simulink model "Rect_fed_NL_load_Single_phase_active_filter"  (R2024b)
settings: Solver=ode4  StartTime=0.0  StopTime=1  FixedStep=1e-6  RelTol=1e-3
undefined symbols (not defined in the file or in its folder): THD
libraries: spsCurrentMeasurementLib x5, spsSeriesRLCBranchLib x5, spsDiodeLib x4, spsMosfetLib x4, spsVoltageMeasurementLib x3, slpidlib x2, spsACVoltageSourceLib x1, spspowerguiLib x1
settings Model: Creator=adity  LastModifiedBy=adity

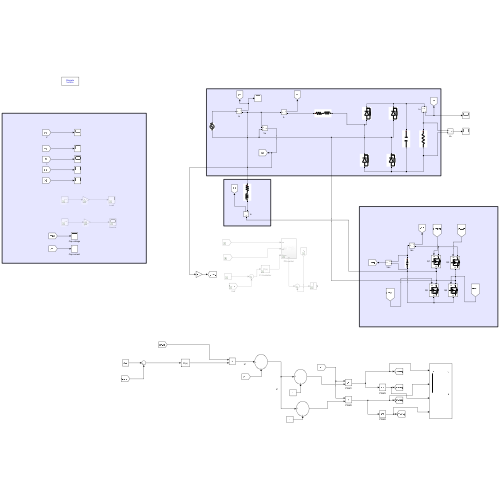
[thumbnail: Simulink's stored preview of the top-level diagram]
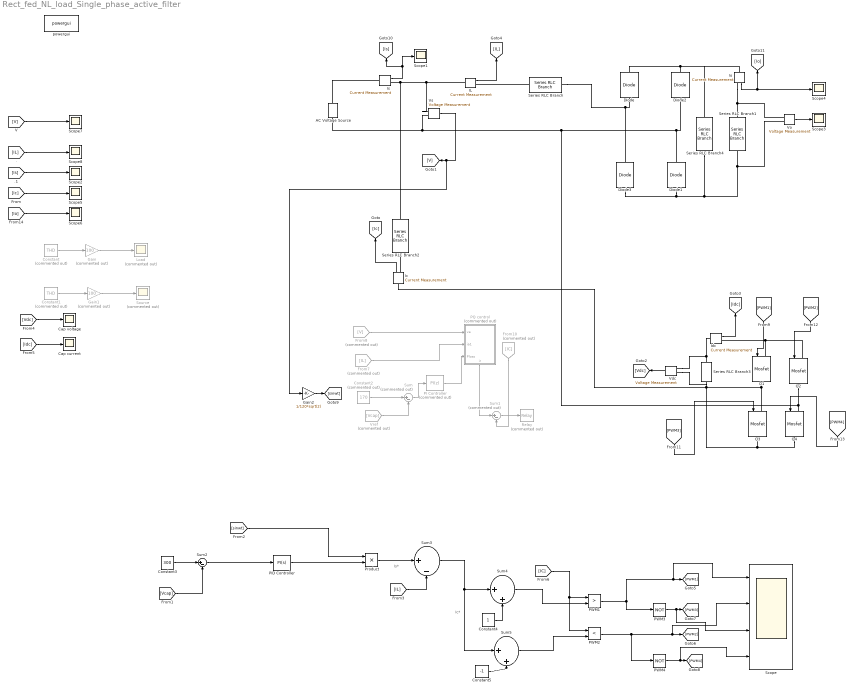
== system Rect_fed_NL_load_Single_phase_active_filter ==
  note: Ic*
  note: Is*
  AC Voltage Source : spsACVoltageSourceLib/AC Voltage Source  Amplitude=120*sqrt(2)  Phase=0  Frequency=60  SampleTime=0  Measurements=None  BusType=swing  Pref=10e3  Qref=0  Qmin=-inf  Qmax=+inf
  Cap current : Scope
  Cap voltage : Scope
  Constant : Constant  Commented=on  Value=THD
  Constant1 : Constant  Commented=on  Value=THD
  Constant2 : Constant  Commented=on  Value=170
  Constant3 : Constant  Value=300
  Constant4 : Constant
  Constant5 : Constant  Value=-1
  Diode{,1..3} (4 alike) : spsDiodeLib/Diode  Ron=0.001  Lon=0  Vf=0.8  IC=0  UseSnubber=0  Rs=500  Cs=250e-9  Measurements=off
  From10 : From  Commented=on  GotoTag=IC
  From7 : From  Commented=on  GotoTag=IL
  From8 : From  Commented=on  GotoTag=V
  Gain : Gain  Commented=on  Gain=100
  Gain1 : Gain  Commented=on  Gain=100
  Gain2 : Gain  Gain=1/120*sqrt(2)
  IL : spsCurrentMeasurementLib/Current Measurement  PhasorSimulation=off  OutputType=Complex  PSBequivalent=0
  Ic : spsCurrentMeasurementLib/Current Measurement  PhasorSimulation=off  OutputType=Complex  PSBequivalent=0
  Idc : spsCurrentMeasurementLib/Current Measurement  PhasorSimulation=off  OutputType=Complex  PSBequivalent=0
  Io : spsCurrentMeasurementLib/Current Measurement  PhasorSimulation=off  OutputType=Complex  PSBequivalent=0
  Is : spsCurrentMeasurementLib/Current Measurement  PhasorSimulation=off  OutputType=Complex  PSBequivalent=0
  Load : Scope  Commented=on
  PI Controller : slpidlib/PID Controller  Commented=on  Controller=PI  Form=Parallel  TimeDomain=Discrete-time  UseExternalTs=off  SampleTime=-1  IntegratorMethod=Forward Euler  FilterMethod=Forward Euler  ControllerParametersSource=internal  P=0.425  I=0.4  UseKiTs=off  D=0  UseExternalDerivativeSource=off  N=100  UseFilter=on  TunerSelectOption=Transfer Function Based (PID Tuner App)  InitialConditionSource=internal  InitialConditionForIntegrator=0  InitialConditionForFilter=0  DifferentiatorICPrevScaledInput=0  ExternalReset=none  TrackingMode=off  Kt=1  LimitOutput=off  SatLimitsSource=internal  UpperSaturationLimit=inf  LowerSaturationLimit=-inf  LinearizeAsGain=on  AntiWindupMode=none  Kb=1  LimitIntegrator=off  UpperIntegratorSaturationLimit=inf  LowerIntegratorSaturationLimit=-inf  POutMin=[]  POutMax=[]  IOutMin=[]  IOutMax=[]  DOutMin=[]  DOutMax=[]  NOutMin=[]  NOutMax=[]  SumOutMin=[]  SumOutMax=[]  SaturationOutMin=[]  SaturationOutMax=[]  PParamMin=[]  PParamMax=[]  IParamMin=[]  IParamMax=[]  DParamMin=[]  DParamMax=[]  NParamMin=[]  NParamMax=[]  KbParamMin=[]  KbParamMax=[]  KtParamMin=[]  KtParamMax=[]  KbOutMin=[]  KbOutMax=[]  KtOutMin=[]  KtOutMax=[]  IntegratorOutMin=[]  IntegratorOutMax=[]  FilterOutMin=[]  FilterOutMax=[]  SumI1OutMin=[]  SumI1OutMax=[]  SumI2OutMin=[]  SumI2OutMax=[]  SumI3OutMin=[]  SumI3OutMax=[]  SumI4OutMin=[]  SumI4OutMax=[]  SumDOutMin=[]  SumDOutMax=[]  DifferentiatorOutMin=[]  DifferentiatorOutMax=[]  FilterDiffOutCoefMin=[]  FilterDiffOutCoefMax=[]  ReciprocalOutMin=[]  ReciprocalOutMax=[]  SumDenOutMin=[]  SumDenOutMax=[]  SumNumOutMin=[]  SumNumOutMax=[]  DivideOutMin=[]  DivideOutMax=[]  UdiffTsProdOutMin=[]  UdiffTsProdOutMax=[]  NTsProdOutMin=[]  NTsProdOutMax=[]  UintegralTsProdOutMin=[]  UintegralTsProdOutMax=[]  UngainTsProdOutMin=[]  UngainTsProdOutMax=[]  ClampingZeroOutDataTypeStr=Inherit: Inherit via back propagation  ClampingZeroOutMin=[]  ClampingZeroOutMax=[]  FilterDenConstantOutDataTypeStr=Inherit: Inherit via back propagation  FilterDenConstantOutMin=[]  FilterDenConstantOutMax=[]  PCopyOutDataTypeStr=Inherit: Inherit via back propagation  PCopyOutMin=[]  PCopyOutMax=[]  NCopyOutDataTypeStr=Inherit: Inherit via back propagation  NCopyOutMin=[]  NCopyOutMax=[]  IntegratorContinuousStateAttributes=''  IntegratorStateMustResolveToSignalObject=off  IntegratorRTWStateStorageClass=Auto  FilterContinuousStateAttributes=''  FilterStateMustResolveToSignalObject=off  FilterRTWStateStorageClass=Auto  ParallelPVariant=InternalParameters  IdealPVariant=Disabled  IVariant=InternalParameters  DVariant=Disabled  IntegratorVariant=Discrete  SatVariant=Disabled  AWVariant=Passthrough  PCopyVariant=Disabled  TRVariant=Disabled  FdbkBlocksVariant=Forward  IdealPFdbkVariant=Disabled  SatFdbkVariant=Disabled  DerivativeFilterVariant=Disabled  NVariant=Disabled  NCopyVariant=Disabled_SignalSpec  FilterICVariant=Disabled  IntegratorICVariant=InternalICs  ExternalResetVariant=Disabled  TRSumVariant=Passthrough  SumFdbkVariant=Disabled  SumVariant=Sum_PI  TsampFilterVariant=InternalTs  TsampNgainVariant=Passthrough  TsampIntegralVariant=Disabled_SignalSpec  ExternalSaturationOutDataTypeStr=Inherit: Same as second input  DerivativeSourceVariant=Disabled  PreIntVariant=InternalPreInt
  PID Controller : slpidlib/PID Controller  Controller=PI  Form=Parallel  TimeDomain=Continuous-time  UseExternalTs=off  SampleTime=-1  IntegratorMethod=Forward Euler  FilterMethod=Forward Euler  ControllerParametersSource=internal  P=0.425  I=0.4  UseKiTs=off  D=0  UseExternalDerivativeSource=off  N=100  UseFilter=on  TunerSelectOption=Transfer Function Based (PID Tuner App)  InitialConditionSource=internal  InitialConditionForIntegrator=0  InitialConditionForFilter=0  DifferentiatorICPrevScaledInput=0  ExternalReset=none  TrackingMode=off  Kt=1  LimitOutput=off  SatLimitsSource=internal  UpperSaturationLimit=inf  LowerSaturationLimit=-inf  LinearizeAsGain=on  AntiWindupMode=none  Kb=1  LimitIntegrator=off  UpperIntegratorSaturationLimit=inf  LowerIntegratorSaturationLimit=-inf  POutMin=[]  POutMax=[]  IOutMin=[]  IOutMax=[]  DOutMin=[]  DOutMax=[]  NOutMin=[]  NOutMax=[]  SumOutMin=[]  SumOutMax=[]  SaturationOutMin=[]  SaturationOutMax=[]  PParamMin=[]  PParamMax=[]  IParamMin=[]  IParamMax=[]  DParamMin=[]  DParamMax=[]  NParamMin=[]  NParamMax=[]  KbParamMin=[]  KbParamMax=[]  KtParamMin=[]  KtParamMax=[]  KbOutMin=[]  KbOutMax=[]  KtOutMin=[]  KtOutMax=[]  IntegratorOutMin=[]  IntegratorOutMax=[]  FilterOutMin=[]  FilterOutMax=[]  SumI1OutMin=[]  SumI1OutMax=[]  SumI2OutMin=[]  SumI2OutMax=[]  SumI3OutMin=[]  SumI3OutMax=[]  SumI4OutMin=[]  SumI4OutMax=[]  SumDOutMin=[]  SumDOutMax=[]  DifferentiatorOutMin=[]  DifferentiatorOutMax=[]  FilterDiffOutCoefMin=[]  FilterDiffOutCoefMax=[]  ReciprocalOutMin=[]  ReciprocalOutMax=[]  SumDenOutMin=[]  SumDenOutMax=[]  SumNumOutMin=[]  SumNumOutMax=[]  DivideOutMin=[]  DivideOutMax=[]  UdiffTsProdOutMin=[]  UdiffTsProdOutMax=[]  NTsProdOutMin=[]  NTsProdOutMax=[]  UintegralTsProdOutMin=[]  UintegralTsProdOutMax=[]  UngainTsProdOutMin=[]  UngainTsProdOutMax=[]  ClampingZeroOutDataTypeStr=Inherit: Inherit via back propagation  ClampingZeroOutMin=[]  ClampingZeroOutMax=[]  FilterDenConstantOutDataTypeStr=Inherit: Inherit via back propagation  FilterDenConstantOutMin=[]  FilterDenConstantOutMax=[]  PCopyOutDataTypeStr=Inherit: Inherit via back propagation  PCopyOutMin=[]  PCopyOutMax=[]  NCopyOutDataTypeStr=Inherit: Inherit via back propagation  NCopyOutMin=[]  NCopyOutMax=[]  IntegratorContinuousStateAttributes=''  IntegratorStateMustResolveToSignalObject=off  IntegratorRTWStateStorageClass=Auto  FilterContinuousStateAttributes=''  FilterStateMustResolveToSignalObject=off  FilterRTWStateStorageClass=Auto  ParallelPVariant=InternalParameters  IdealPVariant=Disabled  IVariant=InternalParameters  DVariant=Disabled  IntegratorVariant=Continuous  SatVariant=Disabled  AWVariant=Passthrough  PCopyVariant=Disabled  TRVariant=Disabled  FdbkBlocksVariant=Forward  IdealPFdbkVariant=Disabled  SatFdbkVariant=Disabled  DerivativeFilterVariant=Disabled  NVariant=Disabled  NCopyVariant=Disabled_SignalSpec  FilterICVariant=Disabled  IntegratorICVariant=InternalICs  ExternalResetVariant=Disabled  TRSumVariant=Passthrough  SumFdbkVariant=Disabled  SumVariant=Sum_PI  TsampFilterVariant=InternalTs  TsampNgainVariant=Passthrough  TsampIntegralVariant=Disabled_SignalSpec  ExternalSaturationOutDataTypeStr=Inherit: Same as second input  DerivativeSourceVariant=Disabled  PreIntVariant=InternalPreInt
  PQ control : Subsystem  Commented=on
      settings: PortSchema="{\"entries\":[{\"content\":{\"sides\":[{\"content\":{\"connectorIds\":[\"In1\",\"In2\",\"In3\"]},\"type\":\"ConnectorPlacement.EquallySpacedRectSide\",\"uuid\":\"c4ed8da9-4339-446b-b803-e8d044cfe926\"},{\"content\":{\"side\":\"RIGHT\"},\"type\":\"ConnectorPlacement.EquallySpacedRectSide\",\"uuid\":\"bd912bfd-ece0-41f3-bab8-21097327688e\"},{\"content\":{\"side\":\"TOP\"},\"type\":\"ConnectorPlacement.EquallySpacedRectSide\",\"uuid\":\"4af82050-6866-4203-a341-3453420f7b72\"},{\"content\":{\"connectorIds\":[\"Out1\"],\"side\":\"BOTTOM\"},\"type\":\"ConnectorPlacement.EquallySpacedRectSide\",\"uuid\":\"e95495c7-7c76-4815-880c-dfa2352730f2\"}]},\"type\":\"ConnectorPlacement.EquallySpacedConnector\",\"uuid\":\"b0fd21c7-50e4-4fd4-87d3-2547b4dd8876\"}],\"packageUris\":[\"http://schema.mathworks.com/mf0/Connector/R2020b\"],\"version\":\"1.0\"}"
  PWM1 : RelationalOperator  Operator=>  OutDataTypeStr=boolean  RndMeth=Simplest  InputSameDT=off
  PWM2 : RelationalOperator  Operator=<  OutDataTypeStr=boolean  RndMeth=Simplest  InputSameDT=off
  PWM3 : Logic  Operator=NOT  AllPortsSameDT=off  OutDataTypeStr=boolean
  PWM4 : Logic  Operator=NOT  AllPortsSameDT=off  OutDataTypeStr=boolean
  Product : Product
  Q{1..4} (4 alike) : spsMosfetLib/Mosfet  Ron=0.1  Lon=0  Rd=0.01  Vfd=0  IC=0  Rs=1e5  Cs=inf  Measurements=off
  Relay : Relay  Commented=on
  Scope : Scope  NumInputPorts=4
  Scope{1..8} (8 alike) : Scope
  Series RLC Branch : spsSeriesRLCBranchLib/Series RLC Branch  LConnTagsString=__new0  RConnTagsString=__new0  BranchType=RL  Resistance=0.25  Inductance=0.25e-3  SetiL0=off  InitialCurrent=0  Capacitance=1e-6  Setx0=off  InitialVoltage=0  Measurements=None
  Series RLC Branch1 : spsSeriesRLCBranchLib/Series RLC Branch  LConnTagsString=__new0  RConnTagsString=__new0  BranchType=R  Resistance=23.2  Inductance=18.006e-3  SetiL0=off  InitialCurrent=0  Capacitance=1e-6  Setx0=off  InitialVoltage=0  Measurements=None
  Series RLC Branch2 : spsSeriesRLCBranchLib/Series RLC Branch  LConnTagsString=__new0  RConnTagsString=__new0  BranchType=RL  Resistance=0.5  Inductance=2.4e-3  SetiL0=off  InitialCurrent=0  Capacitance=1e-6  Setx0=off  InitialVoltage=0  Measurements=None
  Series RLC Branch3 : spsSeriesRLCBranchLib/Series RLC Branch  LConnTagsString=__new0  RConnTagsString=__new0  BranchType=C  Resistance=1  Inductance=1e-3  SetiL0=off  InitialCurrent=0  Capacitance=1000e-6  Setx0=off  InitialVoltage=0  Measurements=None
  Series RLC Branch4 : spsSeriesRLCBranchLib/Series RLC Branch  LConnTagsString=__new0  RConnTagsString=__new0  BranchType=C  Resistance=1  Inductance=1e-3  SetiL0=off  InitialCurrent=0  Capacitance=2200e-6  Setx0=off  InitialVoltage=0  Measurements=None
  Source : Scope  Commented=on
  Sum : Sum  Commented=on  Inputs=|+-
  Sum1 : Sum  Commented=on  Inputs=|+-
  Sum2 : Sum  Inputs=|+-
  Sum3 : Sum  Inputs=|+-
  Sum4 : Sum  Inputs=|++
  Sum5 : Sum  Inputs=|++
  Vdc : spsVoltageMeasurementLib/Voltage Measurement  PhasorSimulation=off  OutputType=Complex  PSBequivalent=0
  Vo : spsVoltageMeasurementLib/Voltage Measurement  PhasorSimulation=off  OutputType=Complex  PSBequivalent=0
  Vref : From  Commented=on  GotoTag=Vcap
  Vs : spsVoltageMeasurementLib/Voltage Measurement  PhasorSimulation=off  OutputType=Complex  PSBequivalent=0
  powergui : spspowerguiLib/powergui  Priority=1  SimulationMode=Discrete  SampleTime=1e-6  frequency=60  Iterations=50  frequencyindice=60  Pbase=100e6  ErrMax=1e-4  UnitsV=kV  UnitsW=MW  buscounter=0  FunctionMessages=off  echomessages=off  EnableUseOfTLC=off  CurrentSourceSwitches=off  DisableSnubberDevices=off  DisableRonSwitches=off  DisableVfSwitches=off  DisplayEquations=off  AutomaticDiscreteSolvers=off  SolverType=Tustin/Backward Euler (TBE)  Interpol=off  ExternalGateDelay=off  methode=off  Ts=100  x0status=blocks  SPID=on  SwTol=0  HookPort=off  NonlinearTolerance=1e-4  nMaxIteration=100  ContinueOnMaxIteration=off  RestoreLinks=warning  ResistiveCurrentMeasurement=off  Frange=[0:2:500]  Ylog=off  Xlog=on  ShowGrid=off  save=off  variable=ZData  structure=0  ZoomFFT=off  StartTime=0.0  cycles=1  DisplayStyle=1  fundamental=60  FreqAxis=off  MaxFrequency=1000  frequencyindicesteady=1  RmsSteady=1  display=off
  wires:
  [V] -> Scope7/1
  Gain/1 -> Load/1
  Gain1/1 -> Source/1
  Constant/1 -> Gain/1
  Constant1/1 -> Gain1/1
  [Vdc] -> Cap voltage/1
  [Idc] -> Cap current/1
  Is/1 -> [Is], Scope1/1
  Ic/1 -> [Ic]
  Constant2/1 -> Sum/1
  Vref/1 -> Sum/2
  Sum/1 -> PI Controller/1
  From10/1 -> Sum1/2
  Vdc/1 -> [Vdc]
  Idc/1 -> [Idc]
  Sum1/1 -> Relay/1
  PI Controller/1 -> PQ control/3(Ploss)
  From8/1 -> PQ control/1(va)
  From7/1 -> PQ control/2(ia1)
  PQ control/1(ir) -> Sum1/1
  IL/1 -> [IL]
  Vo/1 -> Scope3/1
  Io/1 -> [Io], Scope4/1
  [Ic] -> Scope5/1
  [IL] -> Scope8/1
  PWM1/1 -> PWM3/1, Scope/1, [PWM1]
  [Vcap] -> Sum2/2
  [IL] -> Sum3/2
  Product/1 -> Sum3/1
  Sum3/1 -> Sum5/1, Sum4/1
  [sinwt] -> Product/1
  Constant5/1 -> Sum5/2
  Constant3/1 -> Sum2/1
  PWM4/1 -> Scope/4, [PWM4]
  Sum2/1 -> PID Controller/1
  PID Controller/1 -> Product/2
  PWM3/1 -> Scope/3, [PWM3]
  PWM2/1 -> PWM4/1, Scope/2, [PWM2]
  Constant4/1 -> Sum4/2
  Vs/1 -> Gain2/1, [V]
  Gain2/1 -> [sinwt]
  [PWM1] -> Q1/1
  [PWM3] -> Q3/1
  [PWM4] -> Q4/1
  [PWM2] -> Q2/1
  [IC] -> PWM2/1, PWM1/1
  Sum4/1 -> PWM1/2
  Sum5/1 -> PWM2/2
  [Is] -> Scope2/1
  [Io] -> Scope6/1
  connections:
  Is/LConn1 -- AC Voltage Source/RConn1
  IL/LConn1 -- Vs/LConn1 -- Series RLC Branch2/LConn1 -- Is/RConn1
  Series RLC Branch/LConn1 -- IL/RConn1
  Series RLC Branch/RConn1 -- Diode/LConn1 -- Diode3/RConn1
  Diode3/LConn1 -- Diode1/LConn1 -- Vo/LConn2 -- Series RLC Branch1/RConn1 -- Series RLC Branch4/RConn1
  Ic/RConn1 -- Series RLC Branch2/RConn1
  Vdc/LConn1 -- Idc/LConn1 -- Series RLC Branch3/LConn1
  Q1/LConn1 -- Q2/LConn1 -- Idc/RConn1
  Series RLC Branch3/RConn1 -- Q4/RConn1 -- Q3/RConn1 -- Vdc/LConn2
  Vs/LConn2 -- AC Voltage Source/LConn1 -- Diode1/RConn1 -- Diode2/LConn1 -- Q2/RConn1 -- Q4/LConn1
  Q1/RConn1 -- Q3/LConn1 -- Ic/LConn1
  Diode/RConn1 -- Io/LConn1 -- Series RLC Branch4/LConn1 -- Diode2/RConn1
  Io/RConn1 -- Vo/LConn1 -- Series RLC Branch1/LConn1

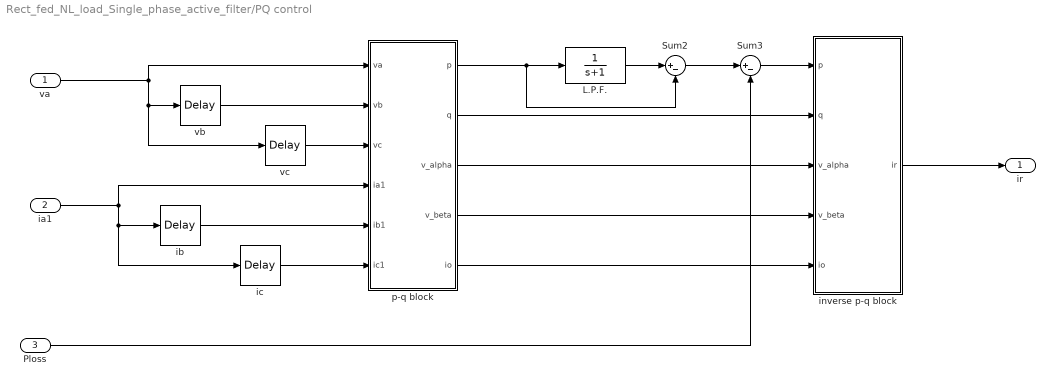
== system Rect_fed_NL_load_Single_phase_active_filter/PQ control ==
  va : Inport
  ia1 : Inport  Port=2
  Ploss : Inport  Port=3
  L.P.F. : TransferFcn  Denominator=[1 1]
  Sum2 : Sum  Inputs=|+-
  Sum3 : Sum  Inputs=|+-
  ib : TransportDelay  DelayTime=(20/3)*0.001
  ic : TransportDelay  DelayTime=(40/3)*0.001
  inverse p-q block : MATLAB Function  TreatAsAtomicUnit=on
  p-q block : MATLAB Function  TreatAsAtomicUnit=on
  vb : TransportDelay  DelayTime=(20/3)*0.001
  vc : TransportDelay  DelayTime=(40/3)*0.001
  ir : Outport
  wires:
  p-q block/5(io) -> inverse p-q block/5(io)
  va/1 -> p-q block/1(va), vc/1, vb/1
  p-q block/1(p) -> Sum2/2, L.P.F./1
  Sum3/1 -> inverse p-q block/1(p)
  vb/1 -> p-q block/2(vb)
  p-q block/4(v_beta) -> inverse p-q block/4(v_beta)
  Sum2/1 -> Sum3/1
  ia1/1 -> ib/1, ic/1, p-q block/4(ia1)
  vc/1 -> p-q block/3(vc)
  p-q block/2(q) -> inverse p-q block/2(q)
  ib/1 -> p-q block/5(ib1)
  inverse p-q block/1(ir) -> ir/1
  p-q block/3(v_alpha) -> inverse p-q block/3(v_alpha)
  ic/1 -> p-q block/6(ic1)
  L.P.F./1 -> Sum2/1
  Ploss/1 -> Sum3/2

== matlab function Rect_fed_NL_load_Single_phase_active_filter/PQ control/inverse p-q block ==
  data: p input; ir output; q input; v_alpha input; v_beta input; io input
function ir = fcn(p,q,v_alpha,v_beta,io)

i_alpha = (v_alpha.*p + v_beta.*q)/(v_alpha.^2 + v_beta.^2);
i_beta = (v_beta.*q - v_alpha.*p)/(v_alpha.^2 + v_beta.^2);
ir = sqrt(2/3)*(io/sqrt(2) + i_alpha);

== matlab function Rect_fed_NL_load_Single_phase_active_filter/PQ control/p-q block ==
  data: va input; p output; vb input; vc input; ia1 input; ib1 input; ic1 input; q output; v_alpha output; v_beta output; io output
function [p,q,v_alpha,v_beta,io] = fcn(va,vb,vc,ia1,ib1,ic1)

v_alpha = (va-vb/2-vc/2)*sqrt(2/3);
v_beta = (vb-vc)/sqrt(2);
io = (ia1+ib1+ic1)/sqrt(3);
i1_alpha = (ia1-ib1/2-ic1/2)*sqrt(2/3);
i1_beta = (ib1-ic1)*sqrt(2);
p = (v_alpha.*i1_alpha) + (v_beta.*i1_beta);
q = (v_beta.*i1_alpha) + (v_alpha.*i1_beta);
